simulink model "TST_CrC_DD"  (R2016b)
settings: Solver=FixedStepDiscrete  StartTime=0.0  StopTime=simTime  FixedStep=sampleTime  RelTol=1e-3
values from neighbouring files (symbols this model uses):
  testCase = 1    [initTST_CrC_DD_001.m]
libraries: simulink x3, UnitTest_Lib x1
settings Model: Creator=xinchangran  LastModifiedBy=xinchangran
settings DebuggingCC: SignalRangeChecking=error

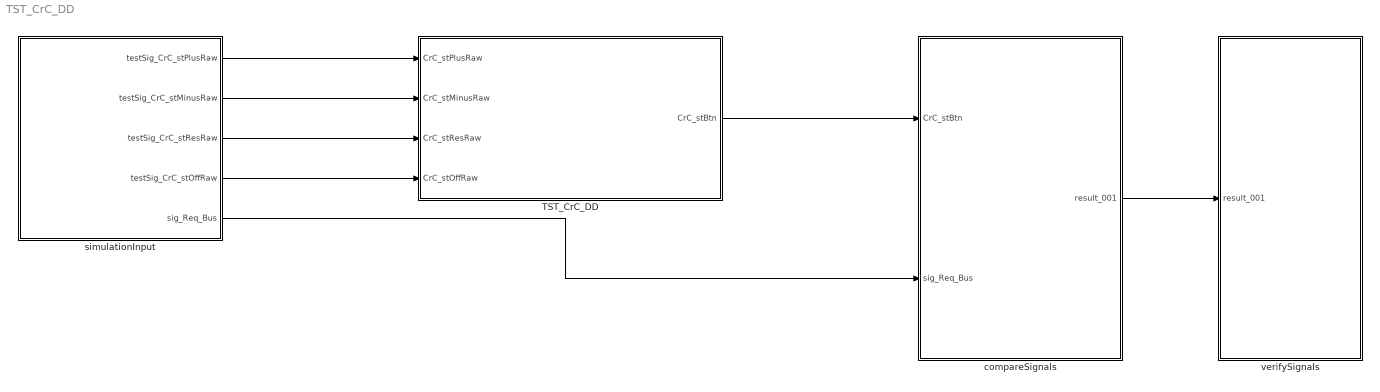
== system TST_CrC_DD ==
  TST_CrC_DD : Subsystem
  compareSignals : Subsystem
  simulationInput : Subsystem
  verifySignals : Subsystem
  wires:
  simulationInput/1(testSig_CrC_stPlusRaw) -> TST_CrC_DD/1(CrC_stPlusRaw)
  simulationInput/2(testSig_CrC_stMinusRaw) -> TST_CrC_DD/2(CrC_stMinusRaw)
  simulationInput/3(testSig_CrC_stResRaw) -> TST_CrC_DD/3(CrC_stResRaw)
  simulationInput/4(testSig_CrC_stOffRaw) -> TST_CrC_DD/4(CrC_stOffRaw)
  TST_CrC_DD/1(CrC_stBtn) -> compareSignals/1(CrC_stBtn)
  simulationInput/5(sig_Req_Bus) -> compareSignals/2(sig_Req_Bus)
  compareSignals/1(result_001) -> verifySignals/1(result_001)

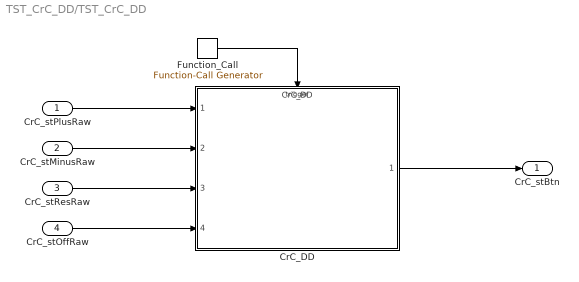
== system TST_CrC_DD/TST_CrC_DD ==
  CrC_stPlusRaw : Inport
  CrC_stMinusRaw : Inport  Port=2
  CrC_stResRaw : Inport  Port=3
  CrC_stOffRaw : Inport  Port=4
  CrC_DD : ModelReference  ModelNameDialog=CrC_DD  SimulationMode=Normal  ModelReferenceVersion=1.34  TriggerPortName=function  TriggerPortTriggerType=function-call  TriggerPortStatesWhenEnabling=held
  Function_Call : simulink/Ports & Subsystems/Function-Call Generator  sample_time=sampleTime  numberOfIterations=1
  CrC_stBtn : Outport
  wires:
  Function_Call/1 -> CrC_DD/Trigger
  CrC_stPlusRaw/1 -> CrC_DD/1
  CrC_stMinusRaw/1 -> CrC_DD/2
  CrC_stResRaw/1 -> CrC_DD/3
  CrC_stOffRaw/1 -> CrC_DD/4
  CrC_DD/1 -> CrC_stBtn/1

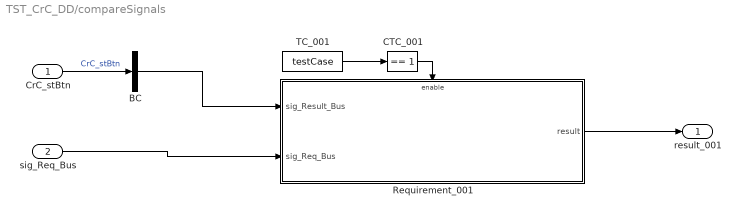
== system TST_CrC_DD/compareSignals ==
  CrC_stBtn : Inport
  sig_Req_Bus : Inport  Port=2
  BC : BusCreator  Inputs=1
  CTC_001 : simulink/Logic and Bit Operations/Compare To Constant  relop===  const=1  OutDataTypeStr=boolean
  Requirement_001 : Subsystem
  TC_001 : Constant  Value=testCase
  result_001 : Outport
  wires:
  CrC_stBtn/1 -> BC/1  "CrC_stBtn"
  TC_001/1 -> CTC_001/1
  CTC_001/1 -> Requirement_001/Enable
  sig_Req_Bus/1 -> Requirement_001/2(sig_Req_Bus)
  BC/1 -> Requirement_001/1(sig_Result_Bus)
  Requirement_001/1(result) -> result_001/1

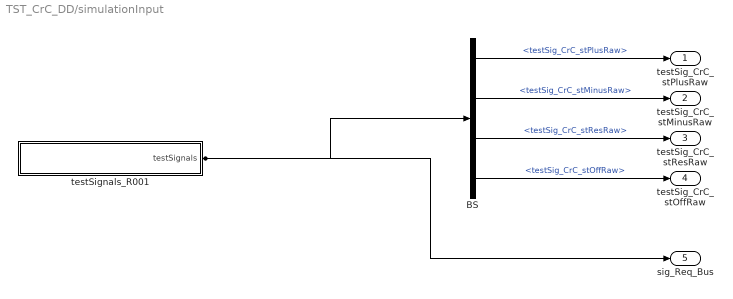
== system TST_CrC_DD/simulationInput ==
  BS : BusSelector  OutputSignals=testSig_CrC_stPlusRaw,testSig_CrC_stMinusRaw,testSig_CrC_stResRaw,testSig_CrC_stOffRaw
  testSignals_R001 : Subsystem
  testSig_CrC_stPlusRaw : Outport
  testSig_CrC_stMinusRaw : Outport  Port=2
  testSig_CrC_stResRaw : Outport  Port=3
  testSig_CrC_stOffRaw : Outport  Port=4
  sig_Req_Bus : Outport  Port=5
  wires:
  BS/1 -> testSig_CrC_stPlusRaw/1  "<testSig_CrC_stPlusRaw>"
  BS/2 -> testSig_CrC_stMinusRaw/1  "<testSig_CrC_stMinusRaw>"
  BS/3 -> testSig_CrC_stResRaw/1  "<testSig_CrC_stResRaw>"
  BS/4 -> testSig_CrC_stOffRaw/1  "<testSig_CrC_stOffRaw>"
  testSignals_R001/1(testSignals) -> BS/1, sig_Req_Bus/1

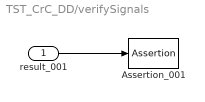
== system TST_CrC_DD/verifySignals ==
  result_001 : Inport
  Assertion_001 : Assertion  Enabled=off
  wires:
  result_001/1 -> Assertion_001/1

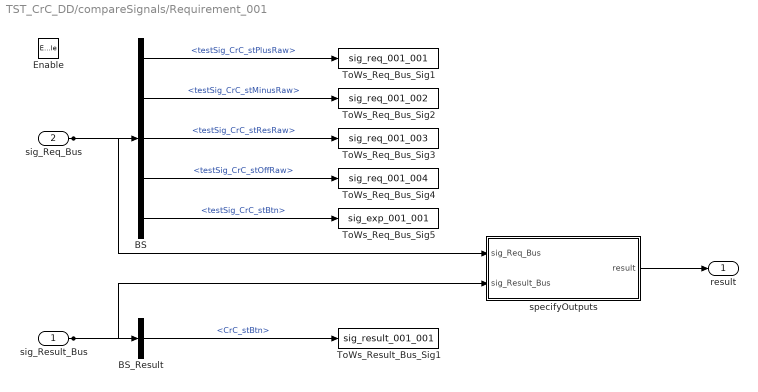
== system TST_CrC_DD/compareSignals/Requirement_001 ==
  sig_Result_Bus : Inport
  sig_Req_Bus : Inport  Port=2
  Enable : EnablePort
  BS : BusSelector  OutputSignals=testSig_CrC_stPlusRaw,testSig_CrC_stMinusRaw,testSig_CrC_stResRaw,testSig_CrC_stOffRaw,testSig_CrC_stBtn
  BS_Result : BusSelector  OutputSignals=CrC_stBtn
  ToWs_Req_Bus_Sig1 : ToWorkspace  VariableName=sig_req_001_001  SaveFormat=Structure With Time
  ToWs_Req_Bus_Sig2 : ToWorkspace  VariableName=sig_req_001_002  SaveFormat=Structure With Time
  ToWs_Req_Bus_Sig3 : ToWorkspace  VariableName=sig_req_001_003  SaveFormat=Structure With Time
  ToWs_Req_Bus_Sig4 : ToWorkspace  VariableName=sig_req_001_004  SaveFormat=Structure With Time
  ToWs_Req_Bus_Sig5 : ToWorkspace  VariableName=sig_exp_001_001  SaveFormat=Structure With Time
  ToWs_Result_Bus_Sig1 : ToWorkspace  VariableName=sig_result_001_001  SaveFormat=Structure With Time
  specifyOutputs : Subsystem
  result : Outport
  wires:
  sig_Req_Bus/1 -> BS/1, specifyOutputs/1(sig_Req_Bus)
  BS/1 -> ToWs_Req_Bus_Sig1/1  "<testSig_CrC_stPlusRaw>"
  BS/2 -> ToWs_Req_Bus_Sig2/1  "<testSig_CrC_stMinusRaw>"
  BS/3 -> ToWs_Req_Bus_Sig3/1  "<testSig_CrC_stResRaw>"
  BS/4 -> ToWs_Req_Bus_Sig4/1  "<testSig_CrC_stOffRaw>"
  BS/5 -> ToWs_Req_Bus_Sig5/1  "<testSig_CrC_stBtn>"
  sig_Result_Bus/1 -> BS_Result/1, specifyOutputs/2(sig_Result_Bus)
  BS_Result/1 -> ToWs_Result_Bus_Sig1/1  "<CrC_stBtn>"
  specifyOutputs/1(result) -> result/1

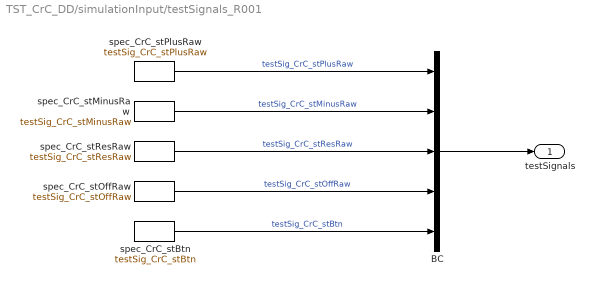
== system TST_CrC_DD/simulationInput/testSignals_R001 ==
  BC : BusCreator  Inputs=5
  spec_CrC_stBtn : FromWorkspace  VariableName=testSig_CrC_stBtn  Interpolate=off  OutputAfterFinalValue=Holding final value
  spec_CrC_stMinusRaw : FromWorkspace  VariableName=testSig_CrC_stMinusRaw  Interpolate=off  OutputAfterFinalValue=Holding final value
  spec_CrC_stOffRaw : FromWorkspace  VariableName=testSig_CrC_stOffRaw  Interpolate=off  OutputAfterFinalValue=Holding final value
  spec_CrC_stPlusRaw : FromWorkspace  VariableName=testSig_CrC_stPlusRaw  Interpolate=off  OutputAfterFinalValue=Holding final value
  spec_CrC_stResRaw : FromWorkspace  VariableName=testSig_CrC_stResRaw  Interpolate=off  OutputAfterFinalValue=Holding final value
  testSignals : Outport
  wires:
  BC/1 -> testSignals/1
  spec_CrC_stPlusRaw/1 -> BC/1  "testSig_CrC_stPlusRaw"
  spec_CrC_stMinusRaw/1 -> BC/2  "testSig_CrC_stMinusRaw"
  spec_CrC_stResRaw/1 -> BC/3  "testSig_CrC_stResRaw"
  spec_CrC_stOffRaw/1 -> BC/4  "testSig_CrC_stOffRaw"
  spec_CrC_stBtn/1 -> BC/5  "testSig_CrC_stBtn"

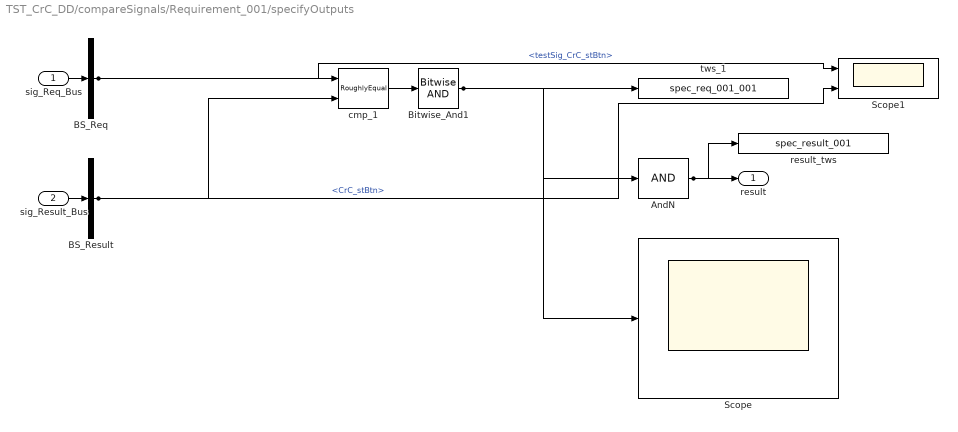
== system TST_CrC_DD/compareSignals/Requirement_001/specifyOutputs ==
  sig_Req_Bus : Inport
  sig_Result_Bus : Inport  Port=2
  AndN : Logic  Inputs=1
  BS_Req : BusSelector  OutputSignals=testSig_CrC_stBtn
  BS_Result : BusSelector  OutputSignals=CrC_stBtn
  Bitwise_And1 : simulink/Logic and Bit Operations/Bitwise Operator  logicop=AND  UseBitMask=off  BitMask=bin2dec('11011001')  BitMaskRealWorld=Stored Integer
  Scope : Scope
  Scope1 : Scope  NumInputPorts=2
  cmp_1 : UnitTest_Lib/RoughlyEqual  slope=0.1
  result_tws : ToWorkspace  VariableName=spec_result_001
  tws_1 : ToWorkspace  VariableName=spec_req_001_001
  result : Outport
  wires:
  sig_Req_Bus/1 -> BS_Req/1
  sig_Result_Bus/1 -> BS_Result/1
  AndN/1 -> result/1, result_tws/1
  BS_Req/1 -> cmp_1/1, Scope1/1  "<testSig_CrC_stBtn>"
  BS_Result/1 -> cmp_1/2, Scope1/2  "<CrC_stBtn>"
  cmp_1/1 -> Bitwise_And1/1
  Bitwise_And1/1 -> tws_1/1, AndN/1, Scope/1
